simulink model "Torque_Mode_OpenLoop"  (R2014a)
settings: Solver=ode5  StartTime=0.0  StopTime=T_f+0.1  FixedStep=0.001  RelTol=1e-3
InitFcn:
  | load('New_Demo')
  | T_f=37;
undefined symbols (not defined in the file or in its folder): Standard_Devices, UDP_Protocol
libraries: simulink x4, rtwinlib x3, slrtlib x1
(part 1 of 2)
settings Model: SimulationMode=external  ExtModeTrigDuration=70000  ExtModeTrigDurationFloating=70000  Creator=user  LastModifiedBy=user
settings HardwareCC: ProdIntDivRoundTo=Zero  ProdEndianess=LittleEndian  ProdHWDeviceType=Generic->32-bit x86 compatible
settings RTWCC: SystemTargetFile=rtwin.tlc  TemplateMakefile=rtwin.tmf  Description=Real-Time Windows Target  ProcessScript=rtwin_make_rtw_hook  RTWCompilerOptimization=On
settings CodeAppCC: MaxIdLength=95
settings RTWinTargetCC: TargetLibSuffix=_rtwin.lib  TargetPreCompLibLocation=C:\Program Files\MATLAB\R2014a\toolbox\rtw\targets\rtwin\lib\win64

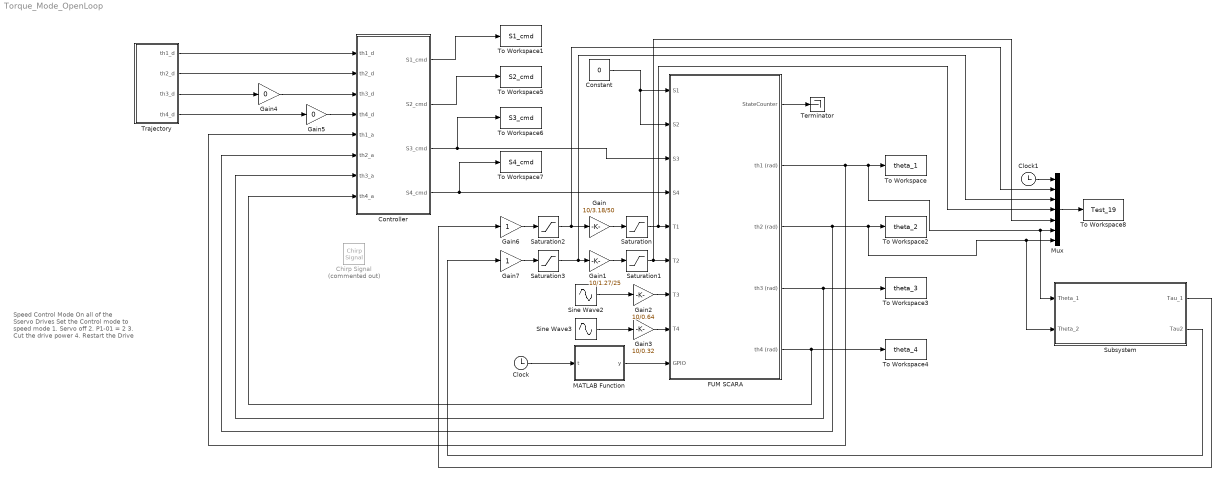
== system Torque_Mode_OpenLoop ==
  note: Speed Control Mode
      | On all of the Sservo Drives Set the
      | Control mode to speed mode
      | 1. Servo off
      | 2. P1-01 = 2
      | 3. Cut the drive power
      | 4. Restart the Drive
  Chirp Signal : simulink/Sources/Chirp Signal  Commented=on  f1=1/2/pi  T=T_f  f2=5/2/pi
  Clock : Clock
      settings: Decimation=20
  Clock1 : Clock
  Constant : Constant  Value=0
  Controller : Subsystem
  FUM SCARA : Subsystem
  Gain : Gain  Gain=10/3.18/50
  Gain1 : Gain  Gain=10/1.27/25
  Gain2 : Gain  Gain=10/0.64
  Gain3 : Gain  Gain=10/0.32
  Gain4 : Gain  Gain=0
  Gain5 : Gain  Gain=0
  Gain6 : Gain
  Gain7 : Gain
  MATLAB Function : MATLAB Function  TreatAsAtomicUnit=on
  Mux : Mux  Inputs=7
  Saturation : Saturate  UpperLimit=5  LowerLimit=-5
  Saturation1 : Saturate  UpperLimit=5  LowerLimit=-5
  Saturation2 : Saturate  UpperLimit=30  LowerLimit=-30
  Saturation3 : Saturate  UpperLimit=10  LowerLimit=-10
  Sine Wave2 : Sin  Amplitude=0  SampleTime=0
  Sine Wave3 : Sin  Amplitude=0  SampleTime=0
  Subsystem : Subsystem
  Terminator : Terminator
  To Workspace : ToWorkspace  VariableName=theta_1  SampleTime=-1
  To Workspace1 : ToWorkspace  VariableName=S1_cmd  SampleTime=-1
  To Workspace2 : ToWorkspace  VariableName=theta_2  SampleTime=-1
  To Workspace3 : ToWorkspace  VariableName=theta_3  SampleTime=-1
  To Workspace4 : ToWorkspace  VariableName=theta_4  SampleTime=-1
  To Workspace5 : ToWorkspace  VariableName=S2_cmd  SampleTime=-1
  To Workspace6 : ToWorkspace  VariableName=S3_cmd  SampleTime=-1
  To Workspace7 : ToWorkspace  VariableName=S4_cmd  SampleTime=-1
  To Workspace8 : ToWorkspace  VariableName=Test_19  SampleTime=-1
  Trajectory : Subsystem
  wires:
  FUM SCARA/1(StateCounter) -> Terminator/1
  Trajectory/1(th1_d) -> Controller/1(th1_d)
  Trajectory/2(th2_d) -> Controller/2(th2_d)
  Trajectory/3(th3_d) -> Gain4/1
  Trajectory/4(th4_d) -> Gain5/1
  FUM SCARA/5(th4 (rad)) -> Controller/8(th4_a), To Workspace4/1
  FUM SCARA/4(th3 (rad)) -> Controller/7(th3_a), To Workspace3/1
  FUM SCARA/3(th2 (rad)) -> Controller/6(th2_a), Subsystem/2(Theta_2), Mux/7, To Workspace2/1
  FUM SCARA/2(th1 (rad)) -> Controller/5(th1_a), Subsystem/1(Theta_1), Mux/6, To Workspace/1
  Clock/1 -> MATLAB Function/1(t)
  MATLAB Function/1(y) -> FUM SCARA/9(GPIO)
  Controller/1(S1_cmd) -> To Workspace1/1
  Controller/2(S2_cmd) -> To Workspace5/1
  Controller/3(S3_cmd) -> To Workspace6/1, FUM SCARA/3(S3)
  Controller/4(S4_cmd) -> FUM SCARA/4(S4), To Workspace7/1
  Constant/1 -> FUM SCARA/2(S2), FUM SCARA/1(S1)
  Sine Wave2/1 -> Gain2/1
  Sine Wave3/1 -> Gain3/1
  Gain/1 -> Saturation/1
  Gain1/1 -> Saturation1/1
  Gain2/1 -> FUM SCARA/7(T3)
  Gain3/1 -> FUM SCARA/8(T4)
  Gain4/1 -> Controller/3(th3_d)
  Gain5/1 -> Controller/4(th4_d)
  Gain6/1 -> Saturation2/1
  Gain7/1 -> Saturation3/1
  Saturation/1 -> Mux/4, FUM SCARA/5(T1)
  Saturation1/1 -> FUM SCARA/6(T2), Mux/5
  Clock1/1 -> Mux/1
  Mux/1 -> To Workspace8/1
  Subsystem/2(Tau2) -> Gain7/1
  Subsystem/1(Tau_1) -> Gain6/1
  Saturation2/1 -> Gain/1, Mux/2
  Saturation3/1 -> Mux/3, Gain1/1

== system Torque_Mode_OpenLoop/Controller ==
  th1_d : Inport
  th2_d : Inport  Port=2
  th3_d : Inport  Port=3
  th4_d : Inport  Port=4
  th1_a : Inport  Port=5
  th2_a : Inport  Port=6
  th3_a : Inport  Port=7
  th4_a : Inport  Port=8
  Gain10 : Gain  Gain=0.25  SampleTime=0.001
  Gain16 : Gain  Gain=0.5  SampleTime=0.001
  Gain5 : Gain  Gain=0.5  SampleTime=0.001
  Gain9 : Gain  Gain=0.4  SampleTime=0.001
  Sum{2,5..6,8} (4 alike) : Sum  Inputs=|+-
  S1_cmd : Outport
  S2_cmd : Outport  Port=2
  S3_cmd : Outport  Port=3
  S4_cmd : Outport  Port=4
  wires:
  th2_a/1 -> Sum2/2
  Sum2/1 -> Gain5/1
  th3_a/1 -> Sum5/2
  Sum5/1 -> Gain10/1
  Sum8/1 -> Gain16/1
  th1_a/1 -> Sum6/2
  th4_a/1 -> Sum8/2
  Sum6/1 -> Gain9/1
  Gain16/1 -> S4_cmd/1
  Gain9/1 -> S1_cmd/1
  Gain5/1 -> S2_cmd/1
  Gain10/1 -> S3_cmd/1
  th2_d/1 -> Sum2/1
  th3_d/1 -> Sum5/1
  th1_d/1 -> Sum6/1
  th4_d/1 -> Sum8/1

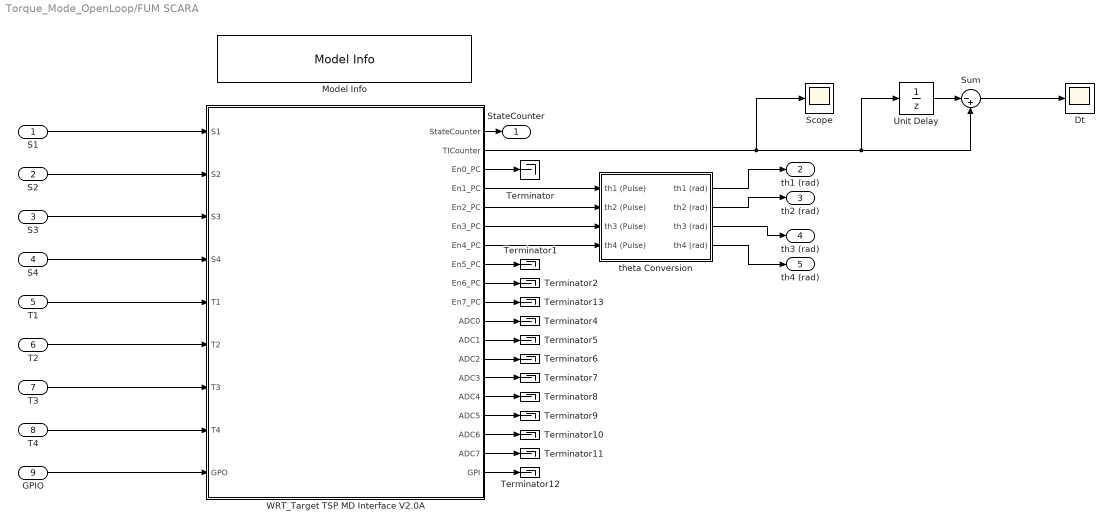
== system Torque_Mode_OpenLoop/FUM SCARA ==
  S1 : Inport
  S2 : Inport  Port=2
  S3 : Inport  Port=3
  S4 : Inport  Port=4
  T1 : Inport  Port=5
  T2 : Inport  Port=6
  T3 : Inport  Port=7
  T4 : Inport  Port=8
  GPIO : Inport  Port=9
  Dt : Scope
      settings: TimeRange=7  YMin=0  YMax=2  SaveName=Dt
  Model Info : simulink/Model-Wide Utilities/Model Info  InitialBlockCM=None  BlockCM=None  Frame=on  DisplayStringWithTags="TSP MD Interface With Windows  Real Time Target"  HorizontalTextAlignment=Center  LeftAlignmentValue=0.5  SourceBlockDiagram=Torque_Mode_OpenLoop  TagMaxNumber=20
  Scope : Scope
      settings: TimeRange=60  YMin=0  YMax=275
  Sum : Sum  Inputs=|-+
  Terminator{,1..2,4..13} (13 alike) : Terminator
  Unit Delay : UnitDelay  SampleTime=-1
  WRT_Target TSP MD Interface V2.0A : Subsystem  mask(TSP MDI Send UDP Packet){SampleTime=0.001, MaxProcTime=T_f*1000, ADC_Mode=8 Single-Ended Inputs, ADC_Range=± 10 V}
      mask prompts: SampleTime "Sample Time"; MaxProcTime "Total Processing Counter"; ADC_Mode "ADC Mode"; ADC_Range "ADC Range"
      mask help: This Block Manage Sending UDP Packet To TSP MDI Board
      mask TypeOptions ADC_Mode: 8 Single-Ended Inputs | 4 Pseudo Differential Inputs | 4 Fully Differential Inputs | Pseudo Differential Inputs
      mask TypeOptions ADC_Range: ± 10 V | ± 5 V | ± 2.5 V | 0-10 V
  theta Conversion : Subsystem
  StateCounter : Outport
  th1 (rad) : Outport  Port=2
  th2 (rad) : Outport  Port=3
  th3 (rad) : Outport  Port=4
  th4 (rad) : Outport  Port=5
  wires:
  WRT_Target TSP MD Interface V2.0A/1(StateCounter) -> StateCounter/1
  WRT_Target TSP MD Interface V2.0A/2(TICounter) -> Scope/1, Unit Delay/1, Sum/2
  theta Conversion/1(th1 (rad)) -> th1 (rad)/1
  theta Conversion/3(th3 (rad)) -> th3 (rad)/1
  theta Conversion/4(th4 (rad)) -> th4 (rad)/1
  Unit Delay/1 -> Sum/1
  WRT_Target TSP MD Interface V2.0A/4(En1_PC) -> theta Conversion/1(th1 (Pulse))
  WRT_Target TSP MD Interface V2.0A/5(En2_PC) -> theta Conversion/2(th2 (Pulse))
  WRT_Target TSP MD Interface V2.0A/6(En3_PC) -> theta Conversion/3(th3 (Pulse))
  WRT_Target TSP MD Interface V2.0A/3(En0_PC) -> Terminator/1
  WRT_Target TSP MD Interface V2.0A/8(En5_PC) -> Terminator1/1
  WRT_Target TSP MD Interface V2.0A/9(En6_PC) -> Terminator2/1
  WRT_Target TSP MD Interface V2.0A/11(ADC0) -> Terminator4/1
  WRT_Target TSP MD Interface V2.0A/12(ADC1) -> Terminator5/1
  WRT_Target TSP MD Interface V2.0A/13(ADC2) -> Terminator6/1
  WRT_Target TSP MD Interface V2.0A/14(ADC3) -> Terminator7/1
  WRT_Target TSP MD Interface V2.0A/15(ADC4) -> Terminator8/1
  WRT_Target TSP MD Interface V2.0A/16(ADC5) -> Terminator9/1
  WRT_Target TSP MD Interface V2.0A/17(ADC6) -> Terminator10/1
  WRT_Target TSP MD Interface V2.0A/18(ADC7) -> Terminator11/1
  WRT_Target TSP MD Interface V2.0A/19(GPI) -> Terminator12/1
  Sum/1 -> Dt/1
  WRT_Target TSP MD Interface V2.0A/7(En4_PC) -> theta Conversion/4(th4 (Pulse))
  WRT_Target TSP MD Interface V2.0A/10("En7_PC ") -> Terminator13/1
  theta Conversion/2(th2 (rad)) -> th2 (rad)/1
  S1/1 -> WRT_Target TSP MD Interface V2.0A/1(S1)
  S2/1 -> WRT_Target TSP MD Interface V2.0A/2(S2)
  S3/1 -> WRT_Target TSP MD Interface V2.0A/3(S3)
  S4/1 -> WRT_Target TSP MD Interface V2.0A/4(S4)
  GPIO/1 -> WRT_Target TSP MD Interface V2.0A/9(GPO)
  T1/1 -> WRT_Target TSP MD Interface V2.0A/5(T1)
  T2/1 -> WRT_Target TSP MD Interface V2.0A/6(T2)
  T3/1 -> WRT_Target TSP MD Interface V2.0A/7(T3)
  T4/1 -> WRT_Target TSP MD Interface V2.0A/8(T4)

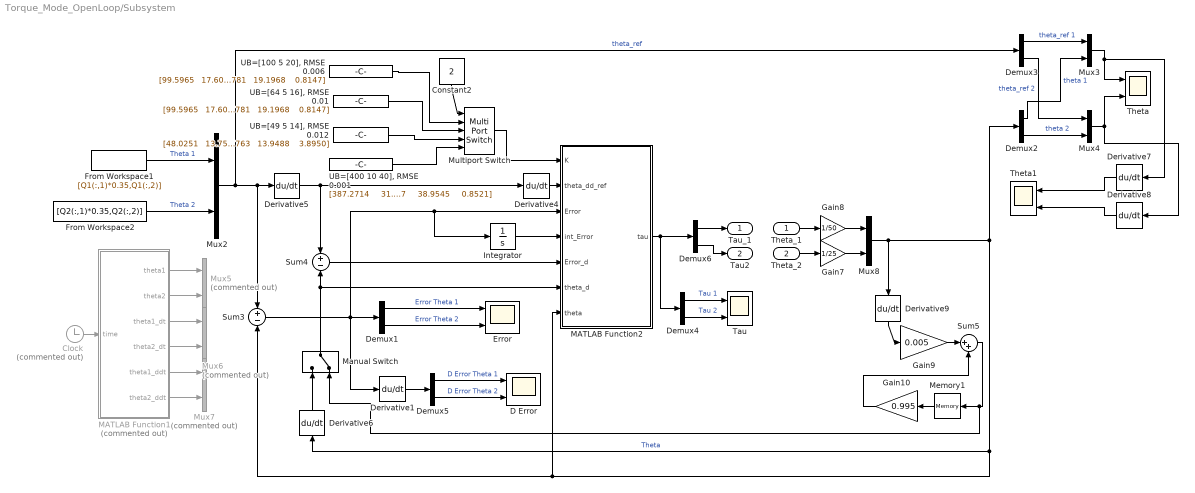
== system Torque_Mode_OpenLoop/Subsystem ==
  Theta_1 : Inport
  Theta_2 : Inport  Port=2
  Clock : Clock  Commented=on
  Constant2 : Constant  Value=2
  D Error : Scope  NumInputPorts=2
      settings: ShowLegends=on  YMin=-0.13078~-0.07305  YMax=0.12037~0.07273  SaveName=ScopeData3
  Demux{1..6} (6 alike) : Demux  Outputs=2
  Derivative{1,4..9} (7 alike) : Derivative
  Error : Scope  NumInputPorts=2
      settings: ShowLegends=on  YMin=-0.00785~-0.01145  YMax=-0.00764~-0.011175  SaveName=ScopeData4
  From Workspace1 : FromWorkspace  VariableName=[Q1(:,1)*0.35,Q1(:,2)]  SampleTime=0
  From Workspace2 : FromWorkspace  VariableName=[Q2(:,1)*0.35,Q2(:,2)]  SampleTime=0
  Gain10 : Gain  Gain=0.995
  Gain7 : Gain  Gain=1/25
  Gain8 : Gain  Gain=1/50
  Gain9 : Gain  Gain=0.005
  Integrator : Integrator
  MATLAB Function1 : MATLAB Function  Commented=on  TreatAsAtomicUnit=on
  MATLAB Function2 : MATLAB Function  TreatAsAtomicUnit=on
  Manual Switch : ManualSwitch  CurrentSetting=0
  Memory1 : Memory
  Multiport Switch : MultiPortSwitch  Inputs=4
  Mux{2..4,8} (4 alike) : Mux  Inputs=2
  Mux5 : Mux  Commented=on  Inputs=2
  Mux6 : Mux  Commented=on  Inputs=2
  Mux7 : Mux  Commented=on  Inputs=2
  Sum3 : Sum  Inputs=+|-
  Sum4 : Sum  Inputs=+|-
  Sum5 : Sum  Inputs=|++
  Tau : Scope  NumInputPorts=2
      settings: ShowLegends=on  YMin=50~0  YMax=550~105  SaveName=ScopeData5
  Theta : Scope  NumInputPorts=2
      settings: ShowLegends=on  YMin=-0.0025~-0.0025  YMax=0.035~0.025  SaveName=ScopeData6
  Theta1 : Scope  NumInputPorts=2
      settings: ShowLegends=on  YMin=-0.49087~-0.49093  YMax=0.49087~0.49136  SaveName=ScopeData7
  "UB=[100 5 20], RMSE 0.006" : Constant  Value="[99.5965   17.6001    3.0916   96.6781   19.1968    0.8147]"
  "UB=[400 10 40], RMSE 0.001" : Constant  Value="[387.2714     31.6242     8.5375     369.6227     38.9545     0.8521]"
  "UB=[49 5 14], RMSE 0.012" : Constant  Value="[48.0251   13.7536    2.4862   48.4763   13.9488    3.8950]"
  "UB=[64 5 16], RMSE 0.01" : Constant  Value="[99.5965   17.6001    3.0916   96.6781   19.1968    0.8147]"
  Tau_1 : Outport
  Tau2 : Outport  Port=2
  wires:
  Sum3/1 -> Demux1/1, Derivative1/1, Integrator/1, MATLAB Function2/3(Error)
  MATLAB Function2/1(tau) -> Demux6/1, Demux4/1
  Mux8/1 -> Derivative9/1, Demux2/1, Derivative6/1, MATLAB Function2/7(theta), Sum3/2  "Theta"
  Sum5/1 -> Manual Switch/2, Memory1/1
  Demux1/2 -> Error/2  "Error Theta 2"
  Demux1/1 -> Error/1  "Error Theta 1"
  Mux3/1 -> Theta/1, Derivative7/1
  Mux4/1 -> Theta/2, Derivative8/1
  Demux2/1 -> Mux3/2  "theta 1"
  Demux3/1 -> Mux3/1  "theta_ref 1"
  Demux2/2 -> Mux4/2  "theta 2"
  Demux3/2 -> Mux4/1  "theta_ref 2"
  Integrator/1 -> MATLAB Function2/4(int_Error)
  Sum4/1 -> MATLAB Function2/5(Error_d)
  From Workspace2/1 -> Mux2/2  "Theta 2"
  From Workspace1/1 -> Mux2/1  "Theta 1"
  Demux4/1 -> Tau/1  "Tau 1"
  Demux4/2 -> Tau/2  "Tau 2"
  Demux5/1 -> D Error/1  "D Error Theta 1"
  Demux5/2 -> D Error/2  "D Error Theta 2"
  Derivative1/1 -> Demux5/1
  "UB=[100 5 20], RMSE 0.006"/1 -> Multiport Switch/2
  Constant2/1 -> Multiport Switch/1
  "UB=[64 5 16], RMSE 0.01"/1 -> Multiport Switch/3
  Clock/1 -> MATLAB Function1/1(time)
  MATLAB Function1/1(theta1) -> Mux5/1
  MATLAB Function1/2(theta2) -> Mux5/2
  MATLAB Function1/5(theta1_ddt) -> Mux7/1
  MATLAB Function1/6(theta2_ddt) -> Mux7/2
  MATLAB Function1/4(theta2_dt) -> Mux6/2
  MATLAB Function1/3(theta1_dt) -> Mux6/1
  "UB=[49 5 14], RMSE 0.012"/1 -> Multiport Switch/4
  Derivative4/1 -> MATLAB Function2/2(theta_dd_ref)
  Mux2/1 -> Derivative5/1, Sum3/1, Demux3/1  "theta_ref"
  Derivative5/1 -> Sum4/1, Derivative4/1
  Derivative7/1 -> Theta1/1
  Derivative8/1 -> Theta1/2
  Demux6/2 -> Tau2/1
  Theta_1/1 -> Gain8/1
  Demux6/1 -> Tau_1/1
  Gain8/1 -> Mux8/1
  Gain7/1 -> Mux8/2
  Theta_2/1 -> Gain7/1
  Memory1/1 -> Gain10/1
  Gain10/1 -> Sum5/2
  Gain9/1 -> Sum5/1
  Manual Switch/1 -> MATLAB Function2/6(theta_d), Sum4/2
  Derivative6/1 -> Manual Switch/1
  Derivative9/1 -> Gain9/1
  Multiport Switch/1 -> MATLAB Function2/1(K)
  "UB=[400 10 40], RMSE 0.001"/1 -> Multiport Switch/5

== system Torque_Mode_OpenLoop/Trajectory ==
  Demux1 : Demux  Outputs=12
  From Workspace : FromWorkspace  VariableName=trajectory  SampleTime=0  OutputAfterFinalValue=Holding final value
  Gain{4,8,15,19} (4 alike) : Gain
  Terminator{1..8} (8 alike) : Terminator
  To Workspace : ToWorkspace  VariableName=th1_d  SampleTime=-1
  To Workspace1 : ToWorkspace  VariableName=th2_d  SampleTime=-1
  To Workspace2 : ToWorkspace  VariableName=th3_d  SampleTime=-1
  To Workspace3 : ToWorkspace  VariableName=th4_d  SampleTime=-1
  th1_d : Outport
  th2_d : Outport  Port=2
  th3_d : Outport  Port=3
  th4_d : Outport  Port=4
  wires:
  Demux1/7 -> Gain15/1
  Demux1/10 -> Gain19/1
  Demux1/4 -> Gain8/1
  Gain15/1 -> To Workspace2/1, th3_d/1
  Gain19/1 -> To Workspace3/1, th4_d/1
  Gain8/1 -> To Workspace1/1, th2_d/1
  Gain4/1 -> To Workspace/1, th1_d/1
  From Workspace/1 -> Demux1/1
  Demux1/1 -> Gain4/1
  Demux1/5 -> Terminator3/1
  Demux1/8 -> Terminator5/1
  Demux1/12 -> Terminator8/1
  Demux1/6 -> Terminator4/1
  Demux1/3 -> Terminator2/1
  Demux1/2 -> Terminator1/1
  Demux1/11 -> Terminator7/1
  Demux1/9 -> Terminator6/1

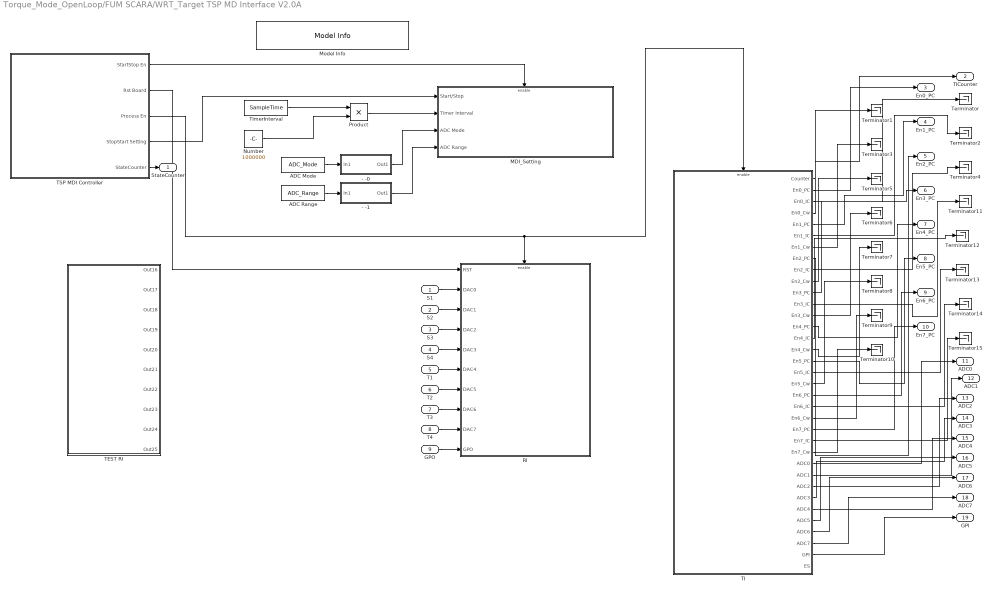
== system Torque_Mode_OpenLoop/FUM SCARA/WRT_Target TSP MD Interface V2.0A ==
  S1 : Inport
  S2 : Inport  Port=2
  S3 : Inport  Port=3
  S4 : Inport  Port=4
  T1 : Inport  Port=5
  T2 : Inport  Port=6
  T3 : Inport  Port=7
  T4 : Inport  Port=8
  GPO : Inport  Port=9
  - -0 : Subsystem
  - -1 : Subsystem
  ADC Mode : Constant  Value=ADC_Mode  SampleTime=-1
  ADC Range : Constant  Value=ADC_Range  SampleTime=-1
  MDI_Setting : Subsystem  TreatAsAtomicUnit=on  mask(Setting UDP Packet Sender){HostMAC=[255 255 255 255 255 255], DeviceMAC=[11 12 13 14 15 16], HostIP1=192, HostIP2=168, HostIP3=1, HostIP4=100, DeviceIP1=192, DeviceIP2=168, DeviceIP3=1, DeviceIP4=22, HostPort=[23000], DevicePort=[23001], SampleTime=SampleTime}
      mask prompts: HostMAC "Host Mac"; DeviceMAC "Device Mac"; HostPort "Host Port"; DevicePort "Device Port"; SampleTime "Sample Time"
      mask help: This Block Genetate And Send UDP Packet To MDI TSP Board For Setting Board
      settings: PropExecContextOutsideSubsystem=on
      mask DialogControl Container10 Prompt: HOST IP
      mask DialogControl Container11 Prompt: DEVICE IP
  Model Info : simulink/Model-Wide Utilities/Model Info  InitialBlockCM=None  BlockCM=None  Frame=on  DisplayStringWithTags=TSP MDI Board With Windows Real Time Target  HorizontalTextAlignment=Center  LeftAlignmentValue=0.5  SourceBlockDiagram=Torque_Mode_OpenLoop  TagMaxNumber=20
  Number : Constant  Value=1000000  SampleTime=-1
  Product : Product
  RI : Subsystem  mask(Receive Informations Packet Generator){En0_e=on, En1_e=on, En2_e=on, En4_e=on, En3_e=on, En5_e=on, En6_e=on, En7_e=on, SampleTime=SampleTime}
      mask prompts: En0_e "Encoder 0 Enable"; En1_e "Encoder 1 Enable"; En2_e "Encoder 2 Enable"; En4_e "Encoder 4 Enable"; En3_e "Encoder 3 Enable"; En5_e "Encoder 5 Enable"; En6_e "Encoder 6 Enable"; En7_e "Encoder 7 Enable"; SampleTime "Sample Time"
      mask DialogControl Control2 Prompt: This Block Generate And Send Receive Informations UDP Packet To MDI TSP Board
  TEST RI : Subsystem
  TI : Subsystem  mask(Receive Information UDP Packet Receiver){SampleTime=SampleTime}
      mask prompts: SampleTime "Sample Time"
      mask help: This Block Receive And Extract Transmit Information UDP Packet From MDI TSP Board
  TSP MDI Controller : Subsystem  mask(TSP MDI Controller){}
      mask help: This Block Controll TSP MDI Board
      mask Help: Set Maximum Count For Time Processing
  Terminator{,1..15} (16 alike) : Terminator
  TimerInterval : Constant  Value=SampleTime  SampleTime=-1
  StateCounter : Outport
  TICounter : Outport  Port=2
  En0_PC : Outport  Port=3
  En1_PC : Outport  Port=4
  En2_PC : Outport  Port=5
  En3_PC : Outport  Port=6
  En4_PC : Outport  Port=7
  En5_PC : Outport  Port=8
  En6_PC : Outport  Port=9
  "En7_PC " : Outport  Port=10
  ADC0 : Outport  Port=11
  ADC1 : Outport  Port=12
  ADC2 : Outport  Port=13
  ADC3 : Outport  Port=14
  ADC4 : Outport  Port=15
  ADC5 : Outport  Port=16
  ADC6 : Outport  Port=17
  ADC7 : Outport  Port=18
  GPI : Outport  Port=19
  wires:
  TI/1(Counter) -> TICounter/1
  TSP MDI Controller/1(StartStop En) -> MDI_Setting/Enable
  TimerInterval/1 -> Product/1
  Number/1 -> Product/2
  Product/1 -> MDI_Setting/2(Timer Interval)
  TI/2(En0_PC) -> En0_PC/1
  TI/5(En1_PC) -> En1_PC/1
  TI/8(En2_PC) -> En2_PC/1
  TI/11(En3_PC) -> En3_PC/1
  TSP MDI Controller/4(StopStart Setting) -> MDI_Setting/1(Start/Stop)
  TSP MDI Controller/3(Process En) -> TI/Enable, RI/Enable
  TSP MDI Controller/5(StateCounter) -> StateCounter/1
  ADC Mode/1 -> - -0/1(In1)
  ADC Range/1 -> - -1/1(In1)
  - -0/1(Out1) -> MDI_Setting/3(ADC Mode)
  - -1/1(Out1) -> MDI_Setting/4(ADC Range)
  TI/26(ADC0) -> ADC0/1
  TI/28(ADC2) -> ADC2/1
  TI/29(ADC3) -> ADC3/1
  TI/30(ADC4) -> ADC4/1
  TI/31(ADC5) -> ADC5/1
  TI/32(ADC6) -> ADC6/1
  TI/33(ADC7) -> ADC7/1
  TI/34(GPI) -> GPI/1
  TI/3(En0_IC) -> Terminator/1
  TI/6(En1_IC) -> Terminator2/1
  TI/9(En2_IC) -> Terminator4/1
  TI/12(En3_IC) -> Terminator11/1
  TI/14(En4_PC) -> En4_PC/1
  TI/15(En4_IC) -> Terminator12/1
  TI/17(En5_PC) -> En5_PC/1
  TI/18(En5_IC) -> Terminator13/1
  TI/20(En6_PC) -> En6_PC/1
  TI/21(En6_IC) -> Terminator14/1
  TI/23(En7_PC) -> "En7_PC "/1
  TI/24(En7_IC) -> Terminator15/1
  TI/4(En0_Cw) -> Terminator1/1
  TI/7(En1_Cw) -> Terminator3/1
  TI/10(En2_Cw) -> Terminator5/1
  TI/13(En3_Cw) -> Terminator6/1
  TI/16(En4_Cw) -> Terminator7/1
  TI/19(En5_Cw) -> Terminator8/1
  TI/22(En6_Cw) -> Terminator9/1
  TI/25(En7_Cw) -> Terminator10/1
  TI/27(ADC1) -> ADC1/1
  GPO/1 -> RI/10(GPO)
  TSP MDI Controller/2(Rst Board) -> RI/1(RST)
  T4/1 -> RI/9(DAC7)
  T3/1 -> RI/8(DAC6)
  T2/1 -> RI/7(DAC5)
  T1/1 -> RI/6(DAC4)
  S1/1 -> RI/2(DAC0)
  S2/1 -> RI/3(DAC1)
  S3/1 -> RI/4(DAC2)
  S4/1 -> RI/5(DAC3)

== system Torque_Mode_OpenLoop/FUM SCARA/theta Conversion ==
  th1 (Pulse) : Inport
  th2 (Pulse) : Inport  Port=2
  th3 (Pulse) : Inport  Port=3
  th4 (Pulse) : Inport  Port=4
  Data Type Conversion{,1..3} (4 alike) : DataTypeConversion  SampleTime=0.001
  Gain{1..2,6,9} (4 alike) : Gain  Gain=1/160000
  Gain{3,7,10,12} (4 alike) : Gain  Gain=2*pi
  Gain{4..5,8,11} (4 alike) : Gain  Gain=-1
  th1 (rad) : Outport
  th2 (rad) : Outport  Port=2
  th3 (rad) : Outport  Port=3
  th4 (rad) : Outport  Port=4
  wires:
  th2 (Pulse)/1 -> Gain2/1
  Gain10/1 -> th4 (rad)/1
  Data Type Conversion3/1 -> Gain11/1
  Gain12/1 -> th1 (rad)/1
  th3 (Pulse)/1 -> Gain6/1
  Data Type Conversion1/1 -> Gain5/1
  th4 (Pulse)/1 -> Gain9/1
  Data Type Conversion2/1 -> Gain8/1
  Gain7/1 -> th3 (rad)/1
  Gain9/1 -> Data Type Conversion3/1
  Gain3/1 -> th2 (rad)/1
  Gain2/1 -> Data Type Conversion1/1
  Gain6/1 -> Data Type Conversion2/1
  Data Type Conversion/1 -> Gain4/1
  Gain1/1 -> Data Type Conversion/1
  th1 (Pulse)/1 -> Gain1/1
  Gain4/1 -> Gain12/1
  Gain5/1 -> Gain3/1
  Gain8/1 -> Gain7/1
  Gain11/1 -> Gain10/1

== system Torque_Mode_OpenLoop/FUM SCARA/WRT_Target TSP MD Interface V2.0A/- -0 ==
  In1 : Inport
  Constant2 : Constant
  Sum : Sum  Inputs=|+-
  Out1 : Outport
  wires:
  In1/1 -> Sum/1
  Sum/1 -> Out1/1
  Constant2/1 -> Sum/2

== system Torque_Mode_OpenLoop/FUM SCARA/WRT_Target TSP MD Interface V2.0A/- -1 ==
  In1 : Inport
  Constant2 : Constant
  Sum : Sum  Inputs=|+-
  Out1 : Outport
  wires:
  In1/1 -> Sum/1
  Sum/1 -> Out1/1
  Constant2/1 -> Sum/2

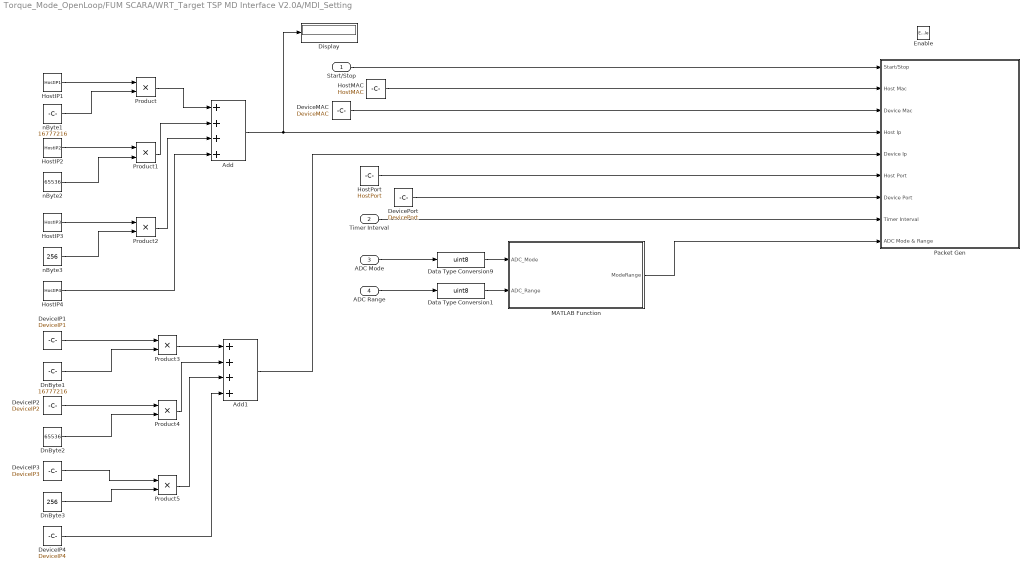
== system Torque_Mode_OpenLoop/FUM SCARA/WRT_Target TSP MD Interface V2.0A/MDI_Setting ==
  Start/Stop : Inport
  Timer Interval : Inport  Port=2
  ADC Mode : Inport  Port=3
  ADC Range : Inport  Port=4
  Enable : EnablePort
  Add : Sum  Inputs=++++
  Add1 : Sum  Inputs=++++
  Data Type Conversion1 : DataTypeConversion  OutDataTypeStr=uint8
  Data Type Conversion9 : DataTypeConversion  OutDataTypeStr=uint8
  DeviceIP1 : Constant  Value=DeviceIP1  SampleTime=-1
  DeviceIP2 : Constant  Value=DeviceIP2  SampleTime=-1
  DeviceIP3 : Constant  Value=DeviceIP3  SampleTime=-1
  DeviceIP4 : Constant  Value=DeviceIP4  SampleTime=-1
  DeviceMAC : Constant  Value=DeviceMAC  SampleTime=-1
  DevicePort : Constant  Value=DevicePort  SampleTime=-1
  Display : Display
  DnByte1 : Constant  Value=16777216
  DnByte2 : Constant  Value=65536  SampleTime=-1
  DnByte3 : Constant  Value=256  SampleTime=-1
  HostIP1 : Constant  Value=HostIP1  SampleTime=-1
  HostIP2 : Constant  Value=HostIP2  SampleTime=-1
  HostIP3 : Constant  Value=HostIP3  SampleTime=-1
  HostIP4 : Constant  Value=HostIP4  SampleTime=-1
  HostMAC : Constant  Value=HostMAC  SampleTime=-1
  HostPort : Constant  Value=HostPort  SampleTime=-1
  MATLAB Function : MATLAB Function  TreatAsAtomicUnit=on
  Packet Gen : Subsystem
  Product{,1..5} (6 alike) : Product
  nByte1 : Constant  Value=16777216
  nByte2 : Constant  Value=65536  SampleTime=-1
  nByte3 : Constant  Value=256  SampleTime=-1
  wires:
  Start/Stop/1 -> Packet Gen/1(Start/Stop)
  HostMAC/1 -> Packet Gen/2(Host Mac)
  DeviceMAC/1 -> Packet Gen/3(Device Mac)
  HostPort/1 -> Packet Gen/6(Host Port)
  DevicePort/1 -> Packet Gen/7(Device Port)
  Timer Interval/1 -> Packet Gen/8(Timer Interval)
  HostIP1/1 -> Product/1
  nByte1/1 -> Product/2
  HostIP2/1 -> Product1/1
  nByte2/1 -> Product1/2
  HostIP3/1 -> Product2/1
  nByte3/1 -> Product2/2
  Product/1 -> Add/1
  Product1/1 -> Add/2
  Product2/1 -> Add/3
  HostIP4/1 -> Add/4
  DeviceIP1/1 -> Product3/1
  DnByte1/1 -> Product3/2
  DeviceIP2/1 -> Product4/1
  DnByte2/1 -> Product4/2
  DeviceIP3/1 -> Product5/1
  DnByte3/1 -> Product5/2
  Product3/1 -> Add1/1
  Product4/1 -> Add1/2
  Product5/1 -> Add1/3
  DeviceIP4/1 -> Add1/4
  Add1/1 -> Packet Gen/5(Device Ip)
  Data Type Conversion9/1 -> MATLAB Function/1(ADC_Mode)
  Data Type Conversion1/1 -> MATLAB Function/2(ADC_Range)
  ADC Mode/1 -> Data Type Conversion9/1
  ADC Range/1 -> Data Type Conversion1/1
  MATLAB Function/1(ModeRange) -> Packet Gen/9(ADC Mode & Range)
  Add/1 -> Display/1, Packet Gen/4(Host Ip)

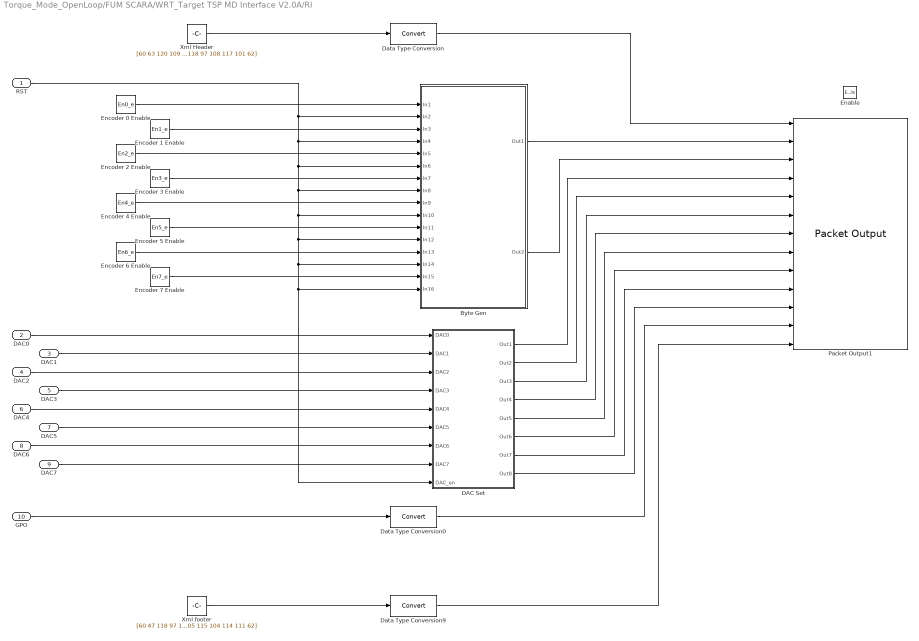
== system Torque_Mode_OpenLoop/FUM SCARA/WRT_Target TSP MD Interface V2.0A/RI ==
  RST : Inport
  DAC0 : Inport  Port=2
  DAC1 : Inport  Port=3
  DAC2 : Inport  Port=4
  DAC3 : Inport  Port=5
  DAC4 : Inport  Port=6
  DAC5 : Inport  Port=7
  DAC6 : Inport  Port=8
  DAC7 : Inport  Port=9
  GPO : Inport  Port=10
  Enable : EnablePort
  Byte Gen : Subsystem
  DAC Set : Subsystem
  Data Type Conversion : DataTypeConversion
  Data Type Conversion0 : DataTypeConversion
  Data Type Conversion9 : DataTypeConversion
  Encoder 0 Enable : Constant  Value=En0_e
  Encoder 1 Enable : Constant  Value=En1_e
  Encoder 2 Enable : Constant  Value=En2_e
  Encoder 3 Enable : Constant  Value=En3_e
  Encoder 4 Enable : Constant  Value=En4_e
  Encoder 5 Enable : Constant  Value=En5_e
  Encoder 6 Enable : Constant  Value=En6_e
  Encoder 7 Enable : Constant  Value=En7_e
  Packet Output1 : rtwinlib/Packet Output  SampleTime=SampleTime  MaxMissedTicks=1000  ShowMissedTicks=off  YieldWhenWaiting=on  DrvName=Standard_Devices/UDP_Protocol  DrvAddress=100  DrvOptions=[3232236031 101]  PacketSize=117  DataTypes={'78*uint8','uint8','uint8','uint16','uint16','uint16','uint16','uint16','uint16','uint16','uint16','uint16','19*uint8'}  ShowReady=off  ShowError=off  PacketID=1  ByteOrder=1  InitialValue=[]  FinalValue=[]
      settings: AttributesFormatString=Standard Devices\nUDP Protocol [64h]
  Xml Header : Constant  Value="[60 63 120 109 108 32 118 101 114 115 105 111 110 61 34  49 46 48 34 63 62 60 116 115 112 105 115 104 114 111 62 60 116 121 112 101 62 114 101 99 101 105 118 101 95 105 110 102 111 60 47 116 121 112 101 62 60 115 105 122 101 62 50 48 60 47 115 105 122 101 62 60 118 97 108 117 101 62]"  LockScale=on
  Xml footer : Constant  Value=[60 47 118 97 108 117 101 62 60 47 116 115 112 105 115 104 114 111 62]
  wires:
  Xml Header/1 -> Data Type Conversion/1
  Xml footer/1 -> Data Type Conversion9/1
  Data Type Conversion/1 -> Packet Output1/1
  Data Type Conversion9/1 -> Packet Output1/13
  Encoder 0 Enable/1 -> Byte Gen/1(In1)
  Encoder 1 Enable/1 -> Byte Gen/3(In3)
  Encoder 2 Enable/1 -> Byte Gen/5(In5)
  Encoder 3 Enable/1 -> Byte Gen/7(In7)
  Encoder 4 Enable/1 -> Byte Gen/9(In9)
  Encoder 6 Enable/1 -> Byte Gen/13(In13)
  Encoder 7 Enable/1 -> Byte Gen/15(In15)
  GPO/1 -> Data Type Conversion0/1
  Data Type Conversion0/1 -> Packet Output1/12
  Byte Gen/1(Out1) -> Packet Output1/2
  Byte Gen/2(Out2) -> Packet Output1/3
  Encoder 5 Enable/1 -> Byte Gen/11(In11)
  DAC0/1 -> DAC Set/1(DAC0)
  DAC1/1 -> DAC Set/2(DAC1)
  DAC2/1 -> DAC Set/3(DAC2)
  DAC3/1 -> DAC Set/4(DAC3)
  DAC4/1 -> DAC Set/5(DAC4)
  DAC5/1 -> DAC Set/6(DAC5)
  DAC6/1 -> DAC Set/7(DAC6)
  DAC7/1 -> DAC Set/8(DAC7)
  RST/1 -> Byte Gen/4(In4), Byte Gen/6(In6), Byte Gen/8(In8), Byte Gen/10(In10), Byte Gen/12(In12), Byte Gen/14(In14), DAC Set/9(DAC_en), Byte Gen/16(In16), Byte Gen/2(In2)
  DAC Set/1(Out1) -> Packet Output1/4
  DAC Set/2(Out2) -> Packet Output1/5
  DAC Set/3(Out3) -> Packet Output1/6
  DAC Set/4(Out4) -> Packet Output1/7
  DAC Set/5(Out5) -> Packet Output1/8
  DAC Set/6(Out6) -> Packet Output1/9
  DAC Set/7(Out7) -> Packet Output1/10
  DAC Set/8(Out8) -> Packet Output1/11

== system Torque_Mode_OpenLoop/FUM SCARA/WRT_Target TSP MD Interface V2.0A/TEST RI ==
  DAC_in0 : Constant  Value=8
  DAC_in1 : Constant  Value=7
  DAC_in2 : Constant  Value=6
  DAC_in3 : Constant  Value=5
  DAC_in4 : Constant  Value=4
  DAC_in5 : Constant  Value=3
  DAC_in6 : Constant  Value=2
  DAC_in7 : Constant
  GPIO : Constant  Value=15  SampleTime=-1
  Rst : Constant  Value=0
  Out16 : Outport
  Out17 : Outport  Port=2
  Out18 : Outport  Port=3
  Out19 : Outport  Port=4
  Out20 : Outport  Port=5
  Out21 : Outport  Port=6
  Out22 : Outport  Port=7
  Out23 : Outport  Port=8
  Out24 : Outport  Port=9
  Out25 : Outport  Port=10
  wires:
  DAC_in4/1 -> Out21/1
  DAC_in6/1 -> Out23/1
  GPIO/1 -> Out25/1
  DAC_in1/1 -> Out18/1
  DAC_in3/1 -> Out20/1
  DAC_in2/1 -> Out19/1
  DAC_in0/1 -> Out17/1
  Rst/1 -> Out16/1
  DAC_in5/1 -> Out22/1
  DAC_in7/1 -> Out24/1

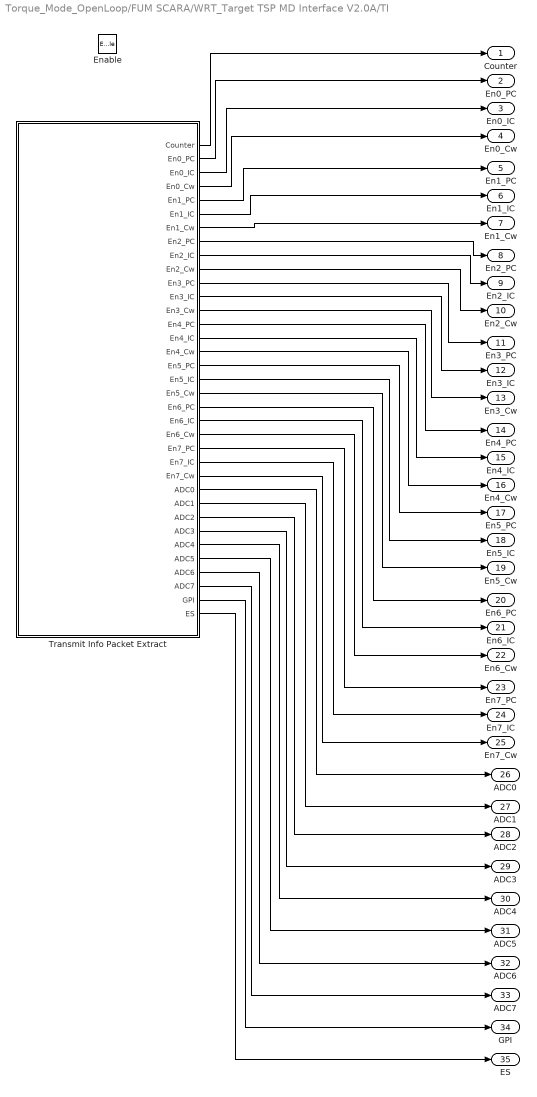
== system Torque_Mode_OpenLoop/FUM SCARA/WRT_Target TSP MD Interface V2.0A/TI ==
  Enable : EnablePort
  Transmit Info Packet Extract : Subsystem
  Counter : Outport
  En0_PC : Outport  Port=2
  En0_IC : Outport  Port=3
  En0_Cw : Outport  Port=4
  En1_PC : Outport  Port=5
  En1_IC : Outport  Port=6
  En1_Cw : Outport  Port=7
  En2_PC : Outport  Port=8
  En2_IC : Outport  Port=9
  En2_Cw : Outport  Port=10
  En3_PC : Outport  Port=11
  En3_IC : Outport  Port=12
  En3_Cw : Outport  Port=13
  En4_PC : Outport  Port=14
  En4_IC : Outport  Port=15
  En4_Cw : Outport  Port=16
  En5_PC : Outport  Port=17
  En5_IC : Outport  Port=18
  En5_Cw : Outport  Port=19
  En6_PC : Outport  Port=20
  En6_IC : Outport  Port=21
  En6_Cw : Outport  Port=22
  En7_PC : Outport  Port=23
  En7_IC : Outport  Port=24
  En7_Cw : Outport  Port=25
  ADC0 : Outport  Port=26
  ADC1 : Outport  Port=27
  ADC2 : Outport  Port=28
  ADC3 : Outport  Port=29
  ADC4 : Outport  Port=30
  ADC5 : Outport  Port=31
  ADC6 : Outport  Port=32
  ADC7 : Outport  Port=33
  GPI : Outport  Port=34
  ES : Outport  Port=35
  wires:
  Transmit Info Packet Extract/1(Counter) -> Counter/1
  Transmit Info Packet Extract/2(En0_PC) -> En0_PC/1
  Transmit Info Packet Extract/3(En0_IC) -> En0_IC/1
  Transmit Info Packet Extract/4(En0_Cw) -> En0_Cw/1
  Transmit Info Packet Extract/5(En1_PC) -> En1_PC/1
  Transmit Info Packet Extract/6(En1_IC) -> En1_IC/1
  Transmit Info Packet Extract/7(En1_Cw) -> En1_Cw/1
  Transmit Info Packet Extract/8(En2_PC) -> En2_PC/1
  Transmit Info Packet Extract/9(En2_IC) -> En2_IC/1
  Transmit Info Packet Extract/10(En2_Cw) -> En2_Cw/1
  Transmit Info Packet Extract/11(En3_PC) -> En3_PC/1
  Transmit Info Packet Extract/12(En3_IC) -> En3_IC/1
  Transmit Info Packet Extract/13(En3_Cw) -> En3_Cw/1
  Transmit Info Packet Extract/14(En4_PC) -> En4_PC/1
  Transmit Info Packet Extract/15(En4_IC) -> En4_IC/1
  Transmit Info Packet Extract/16(En4_Cw) -> En4_Cw/1
  Transmit Info Packet Extract/17(En5_PC) -> En5_PC/1
  Transmit Info Packet Extract/18(En5_IC) -> En5_IC/1
  Transmit Info Packet Extract/19(En5_Cw) -> En5_Cw/1
  Transmit Info Packet Extract/20(En6_PC) -> En6_PC/1
  Transmit Info Packet Extract/21(En6_IC) -> En6_IC/1
  Transmit Info Packet Extract/22(En6_Cw) -> En6_Cw/1
  Transmit Info Packet Extract/23(En7_PC) -> En7_PC/1
  Transmit Info Packet Extract/24(En7_IC) -> En7_IC/1
  Transmit Info Packet Extract/25(En7_Cw) -> En7_Cw/1
  Transmit Info Packet Extract/26(ADC0) -> ADC0/1
  Transmit Info Packet Extract/27(ADC1) -> ADC1/1
  Transmit Info Packet Extract/28(ADC2) -> ADC2/1
  Transmit Info Packet Extract/29(ADC3) -> ADC3/1
  Transmit Info Packet Extract/30(ADC4) -> ADC4/1
  Transmit Info Packet Extract/31(ADC5) -> ADC5/1
  Transmit Info Packet Extract/32(ADC6) -> ADC6/1
  Transmit Info Packet Extract/33(ADC7) -> ADC7/1
  Transmit Info Packet Extract/34(GPI) -> GPI/1
  Transmit Info Packet Extract/35(ES) -> ES/1

== system Torque_Mode_OpenLoop/FUM SCARA/WRT_Target TSP MD Interface V2.0A/TSP MDI Controller ==
  Constant1 : Constant  Value=MaxProcTime  SampleTime=-1
  Counter Limited : simulink/Sources/Counter Limited  uplimit=MaxProcTime  tsamp=SampleTime
  Data Type Conversion : DataTypeConversion
  TSP MDI Control State : Stateflow chart  TreatAsAtomicUnit=on
  StartStop En : Outport
  Rst Board : Outport  Port=2
  Process En : Outport  Port=3
  StopStart Setting : Outport  Port=4
  StateCounter : Outport  Port=5
  wires:
  Counter Limited/1 -> StateCounter/1, Data Type Conversion/1
  TSP MDI Control State/3(ProcessEn) -> Process En/1
  Constant1/1 -> TSP MDI Control State/2(MaxCounter)
  TSP MDI Control State/2(RstBoard) -> Rst Board/1
  TSP MDI Control State/1(StartStopEn) -> StartStop En/1
  TSP MDI Control State/4(StartStopSetting) -> StopStart Setting/1
  Data Type Conversion/1 -> TSP MDI Control State/1(CounterIn)

== system Torque_Mode_OpenLoop/FUM SCARA/WRT_Target TSP MD Interface V2.0A/MDI_Setting/Packet Gen ==
  Start/Stop : Inport
  Host Mac : Inport  Port=2
  Device Mac : Inport  Port=3
  Host Ip : Inport  Port=4
  Device Ip : Inport  Port=5
  Host Port : Inport  Port=6
  Device Port : Inport  Port=7
  Timer Interval : Inport  Port=8
  ADC Mode & Range : Inport  Port=9
  Constant1 : Constant
  Data Type Conversion{,1..10} (11 alike) : DataTypeConversion
  Packet Output : rtwinlib/Packet Output  SampleTime=SampleTime  MaxMissedTicks=1000  ShowMissedTicks=off  YieldWhenWaiting=on  DrvName=Standard_Devices/UDP_Protocol  DrvAddress=100  DrvOptions=[3232236031 101]  PacketSize=126  DataTypes={'126*uint8'}  ShowReady=off  ShowError=off  PacketID=1  ByteOrder=1  InitialValue=[]  FinalValue=[]
      settings: AttributesFormatString=Standard Devices\nUDP Protocol [64h]
  TimeGen : Subsystem
  Udp Setting : slrtlib/UDP/Pack   datatypes={'uint8','uint8','uint8','uint8','uint32','uint32','uint16','uint16','uint32','uint8','uint8'}  byteAlign=1
  Xml Header : Constant  Value=[60 63 120 109 108 32 118 101 114 115 105 111 110 61 34 49 46 48 34 63 62 60 116 115 112 105 115 104 114 111 62 60 116 121 112 101 62 77 68 73 95 115 101 116 116 105 110 103 60 47 116 121 112 101 62 60 115 105 122 101 62 51 48 60 47 115 105 122 101 62 60 118 97 108 117 101 62 ]  SampleTime=-1  LockScale=on
  Xml footer : Constant  Value=[60 47 118 97 108 117 101 62 60 47 116 115 112 105 115 104 114 111 62]  SampleTime=-1
  wires:
  Start/Stop/1 -> Data Type Conversion1/1
  Xml Header/1 -> Data Type Conversion/1
  Data Type Conversion/1 -> Udp Setting/1
  Host Mac/1 -> Data Type Conversion2/1
  Device Mac/1 -> Data Type Conversion3/1
  Host Ip/1 -> Data Type Conversion4/1
  Device Ip/1 -> Data Type Conversion5/1
  Host Port/1 -> Data Type Conversion6/1
  Device Port/1 -> Data Type Conversion7/1
  Timer Interval/1 -> TimeGen/1(value_time)
  ADC Mode & Range/1 -> Data Type Conversion8/1
  Data Type Conversion8/1 -> Udp Setting/10
  Xml footer/1 -> Data Type Conversion9/1
  Data Type Conversion9/1 -> Udp Setting/11
  Data Type Conversion2/1 -> Udp Setting/3
  Data Type Conversion3/1 -> Udp Setting/4
  Data Type Conversion4/1 -> Udp Setting/5
  Data Type Conversion5/1 -> Udp Setting/6
  Data Type Conversion6/1 -> Udp Setting/7
  Data Type Conversion7/1 -> Udp Setting/8
  Data Type Conversion10/1 -> Udp Setting/9
  Data Type Conversion1/1 -> Udp Setting/2
  TimeGen/1(Time_value) -> Data Type Conversion10/1
  Udp Setting/1 -> Packet Output/1

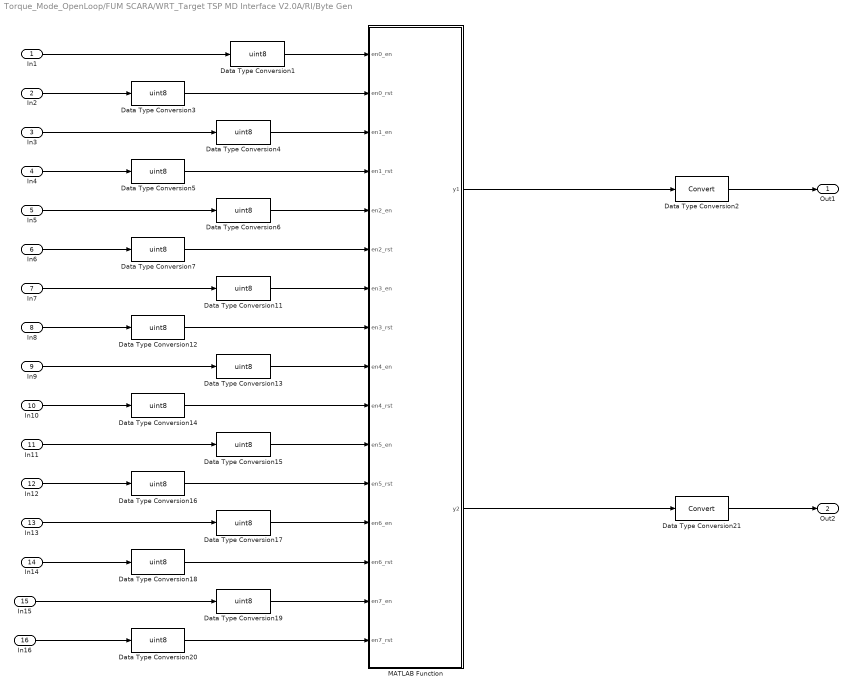
== system Torque_Mode_OpenLoop/FUM SCARA/WRT_Target TSP MD Interface V2.0A/RI/Byte Gen ==
  In1 : Inport
  In2 : Inport  Port=2
  In3 : Inport  Port=3
  In4 : Inport  Port=4
  In5 : Inport  Port=5
  In6 : Inport  Port=6
  In7 : Inport  Port=7
  In8 : Inport  Port=8
  In9 : Inport  Port=9
  In10 : Inport  Port=10
  In11 : Inport  Port=11
  In12 : Inport  Port=12
  In13 : Inport  Port=13
  In14 : Inport  Port=14
  In15 : Inport  Port=15
  In16 : Inport  Port=16
  Data Type Conversion{1,3..7,11..20} (16 alike) : DataTypeConversion  OutDataTypeStr=uint8
  Data Type Conversion2 : DataTypeConversion
  Data Type Conversion21 : DataTypeConversion
  MATLAB Function : MATLAB Function  TreatAsAtomicUnit=on
  Out1 : Outport
  Out2 : Outport  Port=2
  wires:
  In2/1 -> Data Type Conversion3/1
  Data Type Conversion21/1 -> Out2/1
  Data Type Conversion20/1 -> MATLAB Function/16(en7_rst)
  MATLAB Function/1(y1) -> Data Type Conversion2/1
  In11/1 -> Data Type Conversion15/1
  Data Type Conversion15/1 -> MATLAB Function/11(en5_en)
  In14/1 -> Data Type Conversion18/1
  In5/1 -> Data Type Conversion6/1
  Data Type Conversion17/1 -> MATLAB Function/13(en6_en)
  MATLAB Function/2(y2) -> Data Type Conversion21/1
  Data Type Conversion16/1 -> MATLAB Function/12(en5_rst)
  Data Type Conversion18/1 -> MATLAB Function/14(en6_rst)
  Data Type Conversion19/1 -> MATLAB Function/15(en7_en)
  Data Type Conversion1/1 -> MATLAB Function/1(en0_en)
  In10/1 -> Data Type Conversion14/1
  Data Type Conversion11/1 -> MATLAB Function/7(en3_en)
  Data Type Conversion5/1 -> MATLAB Function/4(en1_rst)
  In6/1 -> Data Type Conversion7/1
  Data Type Conversion6/1 -> MATLAB Function/5(en2_en)
  In15/1 -> Data Type Conversion19/1
  In16/1 -> Data Type Conversion20/1
  Data Type Conversion12/1 -> MATLAB Function/8(en3_rst)
  Data Type Conversion4/1 -> MATLAB Function/3(en1_en)
  In9/1 -> Data Type Conversion13/1
  Data Type Conversion7/1 -> MATLAB Function/6(en2_rst)
  Data Type Conversion3/1 -> MATLAB Function/2(en0_rst)
  In4/1 -> Data Type Conversion5/1
  In13/1 -> Data Type Conversion17/1
  In7/1 -> Data Type Conversion11/1
  In8/1 -> Data Type Conversion12/1
  In12/1 -> Data Type Conversion16/1
  In3/1 -> Data Type Conversion4/1
  Data Type Conversion14/1 -> MATLAB Function/10(en4_rst)
  Data Type Conversion13/1 -> MATLAB Function/9(en4_en)
  In1/1 -> Data Type Conversion1/1
  Data Type Conversion2/1 -> Out1/1

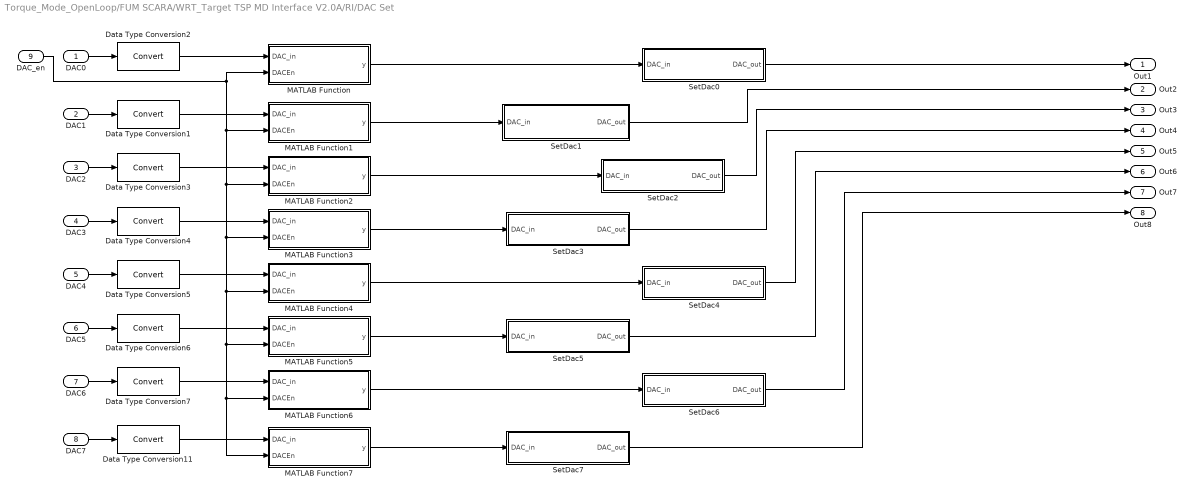
== system Torque_Mode_OpenLoop/FUM SCARA/WRT_Target TSP MD Interface V2.0A/RI/DAC Set ==
  DAC0 : Inport
  DAC1 : Inport  Port=2
  DAC2 : Inport  Port=3
  DAC3 : Inport  Port=4
  DAC4 : Inport  Port=5
  DAC5 : Inport  Port=6
  DAC6 : Inport  Port=7
  DAC7 : Inport  Port=8
  DAC_en : Inport  Port=9
  Data Type Conversion{1..7,11} (8 alike) : DataTypeConversion
  MATLAB Function : MATLAB Function  TreatAsAtomicUnit=on
  MATLAB Function1 : MATLAB Function  TreatAsAtomicUnit=on
  MATLAB Function2 : MATLAB Function  TreatAsAtomicUnit=on
  MATLAB Function3 : MATLAB Function  TreatAsAtomicUnit=on
  MATLAB Function4 : MATLAB Function  TreatAsAtomicUnit=on
  MATLAB Function5 : MATLAB Function  TreatAsAtomicUnit=on
  MATLAB Function6 : MATLAB Function  TreatAsAtomicUnit=on
  MATLAB Function7 : MATLAB Function  TreatAsAtomicUnit=on
  SetDac0 : Subsystem
  SetDac1 : Subsystem
  SetDac2 : Subsystem
  SetDac3 : Subsystem
  SetDac4 : Subsystem
  SetDac5 : Subsystem
  SetDac6 : Subsystem
  SetDac7 : Subsystem
  Out1 : Outport
  Out2 : Outport  Port=2
  Out3 : Outport  Port=3
  Out4 : Outport  Port=4
  Out5 : Outport  Port=5
  Out6 : Outport  Port=6
  Out7 : Outport  Port=7
  Out8 : Outport  Port=8
  wires:
  Data Type Conversion4/1 -> MATLAB Function3/1(DAC_in)
  SetDac0/1(DAC_out) -> Out1/1
  SetDac1/1(DAC_out) -> Out2/1
  SetDac2/1(DAC_out) -> Out3/1
  SetDac3/1(DAC_out) -> Out4/1
  SetDac4/1(DAC_out) -> Out5/1
  SetDac5/1(DAC_out) -> Out6/1
  SetDac6/1(DAC_out) -> Out7/1
  SetDac7/1(DAC_out) -> Out8/1
  MATLAB Function6/1(y) -> SetDac6/1(DAC_in)
  DAC4/1 -> Data Type Conversion5/1
  DAC3/1 -> Data Type Conversion4/1
  DAC7/1 -> Data Type Conversion11/1
  MATLAB Function1/1(y) -> SetDac1/1(DAC_in)
  MATLAB Function4/1(y) -> SetDac4/1(DAC_in)
  DAC6/1 -> Data Type Conversion7/1
  DAC1/1 -> Data Type Conversion1/1
  MATLAB Function7/1(y) -> SetDac7/1(DAC_in)
  DAC_en/1 -> MATLAB Function/2(DACEn), MATLAB Function1/2(DACEn), MATLAB Function2/2(DACEn), MATLAB Function3/2(DACEn), MATLAB Function4/2(DACEn), MATLAB Function5/2(DACEn), MATLAB Function6/2(DACEn), MATLAB Function7/2(DACEn)
  DAC2/1 -> Data Type Conversion3/1
  MATLAB Function5/1(y) -> SetDac5/1(DAC_in)
  MATLAB Function3/1(y) -> SetDac3/1(DAC_in)
  DAC5/1 -> Data Type Conversion6/1
  Data Type Conversion1/1 -> MATLAB Function1/1(DAC_in)
  Data Type Conversion6/1 -> MATLAB Function5/1(DAC_in)
  MATLAB Function/1(y) -> SetDac0/1(DAC_in)
  MATLAB Function2/1(y) -> SetDac2/1(DAC_in)
  Data Type Conversion11/1 -> MATLAB Function7/1(DAC_in)
  Data Type Conversion2/1 -> MATLAB Function/1(DAC_in)
  Data Type Conversion5/1 -> MATLAB Function4/1(DAC_in)
  Data Type Conversion7/1 -> MATLAB Function6/1(DAC_in)
  Data Type Conversion3/1 -> MATLAB Function2/1(DAC_in)
  DAC0/1 -> Data Type Conversion2/1

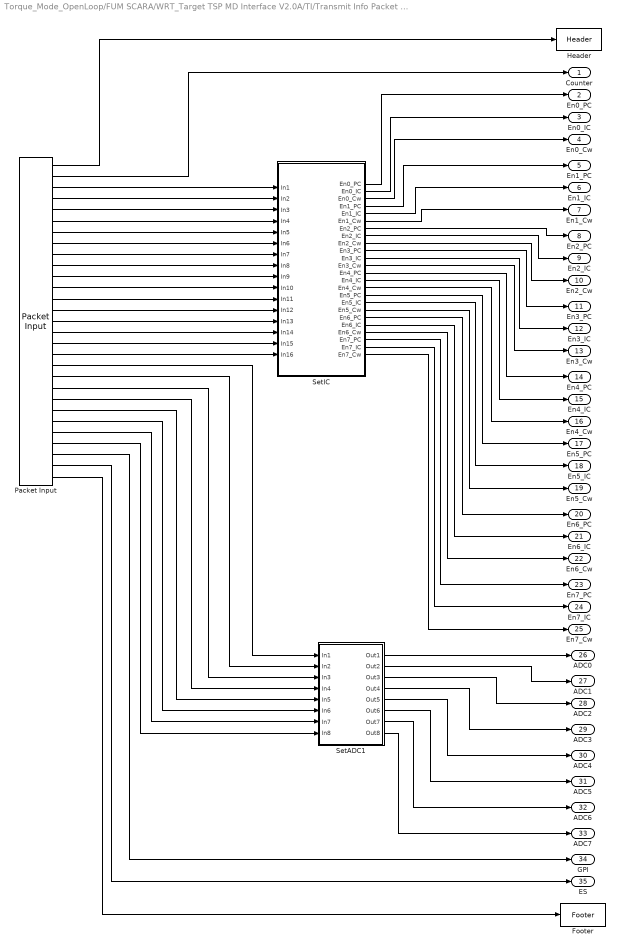
== system Torque_Mode_OpenLoop/FUM SCARA/WRT_Target TSP MD Interface V2.0A/TI/Transmit Info Packet Extract ==
  Footer : ToWorkspace  VariableName=Footer  SaveFormat=Timeseries  SampleTime=-1
  Header : ToWorkspace  VariableName=Header  SaveFormat=Timeseries  SampleTime=-1
  Packet Input : rtwinlib/Packet Input  SampleTime=SampleTime  MaxMissedTicks=1000  ShowMissedTicks=off  YieldWhenWaiting=on  DrvName=Standard_Devices/UDP_Protocol  DrvAddress=23000  DrvOptions=[3232235798 23001]  PacketSize=186  DataTypes="{'81*uint8' 'uint8' 'int32' 'uint32' 'int32' 'uint32' 'int32' 'uint32' 'int32' 'uint32' 'int32' 'uint32' 'int32' 'uint32' 'int32' 'uint32' 'int32' 'uint32' 'int16' 'int16' 'int16' 'int16' 'int16' 'int16' 'int16' 'int16' 'uint32'  'uint8' '19*uint8'}"  ShowReady=off  ShowError=off  PacketID=1  ByteOrder=1  ShowTimestamp=off
      settings: AttributesFormatString=Standard Devices\nUDP Protocol [59D8h]
  SetADC1 : Subsystem
  SetIC : Subsystem
  Counter : Outport
  En0_PC : Outport  Port=2
  En0_IC : Outport  Port=3
  En0_Cw : Outport  Port=4
  En1_PC : Outport  Port=5
  En1_IC : Outport  Port=6
  En1_Cw : Outport  Port=7
  En2_PC : Outport  Port=8
  En2_IC : Outport  Port=9
  En2_Cw : Outport  Port=10
  En3_PC : Outport  Port=11
  En3_IC : Outport  Port=12
  En3_Cw : Outport  Port=13
  En4_PC : Outport  Port=14
  En4_IC : Outport  Port=15
  En4_Cw : Outport  Port=16
  En5_PC : Outport  Port=17
  En5_IC : Outport  Port=18
  En5_Cw : Outport  Port=19
  En6_PC : Outport  Port=20
  En6_IC : Outport  Port=21
  En6_Cw : Outport  Port=22
  En7_PC : Outport  Port=23
  En7_IC : Outport  Port=24
  En7_Cw : Outport  Port=25
  ADC0 : Outport  Port=26
  ADC1 : Outport  Port=27
  ADC2 : Outport  Port=28
  ADC3 : Outport  Port=29
  ADC4 : Outport  Port=30
  ADC5 : Outport  Port=31
  ADC6 : Outport  Port=32
  ADC7 : Outport  Port=33
  GPI : Outport  Port=34
  ES : Outport  Port=35
  wires:
  Packet Input/1 -> Header/1
  Packet Input/26 -> SetADC1/8(In8)
  Packet Input/25 -> SetADC1/7(In7)
  Packet Input/24 -> SetADC1/6(In6)
  Packet Input/23 -> SetADC1/5(In5)
  Packet Input/22 -> SetADC1/4(In4)
  Packet Input/21 -> SetADC1/3(In3)
  Packet Input/20 -> SetADC1/2(In2)
  Packet Input/19 -> SetADC1/1(In1)
  Packet Input/2 -> Counter/1
  SetADC1/8(Out8) -> ADC7/1
  SetADC1/7(Out7) -> ADC6/1
  SetADC1/6(Out6) -> ADC5/1
  SetADC1/5(Out5) -> ADC4/1
  SetADC1/4(Out4) -> ADC3/1
  SetADC1/3(Out3) -> ADC2/1
  SetADC1/2(Out2) -> ADC1/1
  SetADC1/1(Out1) -> ADC0/1
  Packet Input/27 -> GPI/1
  Packet Input/3 -> SetIC/1(In1)
  Packet Input/4 -> SetIC/2(In2)
  Packet Input/5 -> SetIC/3(In3)
  Packet Input/6 -> SetIC/4(In4)
  Packet Input/7 -> SetIC/5(In5)
  Packet Input/8 -> SetIC/6(In6)
  Packet Input/9 -> SetIC/7(In7)
  Packet Input/10 -> SetIC/8(In8)
  Packet Input/11 -> SetIC/9(In9)
  Packet Input/12 -> SetIC/10(In10)
  Packet Input/13 -> SetIC/11(In11)
  Packet Input/14 -> SetIC/12(In12)
  Packet Input/15 -> SetIC/13(In13)
  Packet Input/16 -> SetIC/14(In14)
  Packet Input/17 -> SetIC/15(In15)
  Packet Input/18 -> SetIC/16(In16)
  SetIC/1(En0_PC) -> En0_PC/1
  SetIC/2(En0_IC) -> En0_IC/1
  SetIC/3(En0_Cw) -> En0_Cw/1
  SetIC/4(En1_PC) -> En1_PC/1
  SetIC/5(En1_IC) -> En1_IC/1
  SetIC/6(En1_Cw) -> En1_Cw/1
  SetIC/7(En2_PC) -> En2_PC/1
  SetIC/8(En2_IC) -> En2_IC/1
  SetIC/9(En2_Cw) -> En2_Cw/1
  SetIC/10(En3_PC) -> En3_PC/1
  SetIC/11(En3_IC) -> En3_IC/1
  SetIC/12(En3_Cw) -> En3_Cw/1
  SetIC/13(En4_PC) -> En4_PC/1
  SetIC/14(En4_IC) -> En4_IC/1
  SetIC/15(En4_Cw) -> En4_Cw/1
  SetIC/16(En5_PC) -> En5_PC/1
  SetIC/17(En5_IC) -> En5_IC/1
  SetIC/18(En5_Cw) -> En5_Cw/1
  SetIC/19(En6_PC) -> En6_PC/1
  SetIC/20(En6_IC) -> En6_IC/1
  SetIC/21(En6_Cw) -> En6_Cw/1
  SetIC/22(En7_PC) -> En7_PC/1
  SetIC/23(En7_IC) -> En7_IC/1
  SetIC/24(En7_Cw) -> En7_Cw/1
  Packet Input/29 -> Footer/1
  Packet Input/28 -> ES/1

== system Torque_Mode_OpenLoop/FUM SCARA/WRT_Target TSP MD Interface V2.0A/MDI_Setting/Packet Gen/TimeGen ==
  value_time : Inport
  Constant : Constant  Value=100  SampleTime=-1
  Product : Product
  Time_value : Outport
  wires:
  value_time/1 -> Product/1
  Product/1 -> Time_value/1
  Constant/1 -> Product/2

== system Torque_Mode_OpenLoop/FUM SCARA/WRT_Target TSP MD Interface V2.0A/RI/DAC Set/SetDac0 ==
  DAC_in : Inport
  Add : Sum
  Data Type Conversion0 : DataTypeConversion
  Divide : Product  Inputs=*/
  Divide_numb : Constant  Value=20
  FFFF_numb : Constant  Value=65535
  Product : Product
  Product_numb : Constant  Value=10
  DAC_out : Outport
  wires:
  Divide_numb/1 -> Divide/2
  Product/1 -> Divide/1
  Divide/1 -> Data Type Conversion0/1
  Product_numb/1 -> Add/2
  FFFF_numb/1 -> Product/2
  Add/1 -> Product/1
  DAC_in/1 -> Add/1
  Data Type Conversion0/1 -> DAC_out/1

== system Torque_Mode_OpenLoop/FUM SCARA/WRT_Target TSP MD Interface V2.0A/RI/DAC Set/SetDac1 ==
  DAC_in : Inport
  Add : Sum
  Data Type Conversion0 : DataTypeConversion
  Divide : Product  Inputs=*/
  Divide_numb : Constant  Value=20
  FFFF_numb : Constant  Value=65535
  Product : Product
  Product_numb : Constant  Value=10
  DAC_out : Outport
  wires:
  Divide_numb/1 -> Divide/2
  Product/1 -> Divide/1
  Divide/1 -> Data Type Conversion0/1
  Product_numb/1 -> Add/2
  FFFF_numb/1 -> Product/2
  Add/1 -> Product/1
  DAC_in/1 -> Add/1
  Data Type Conversion0/1 -> DAC_out/1

== system Torque_Mode_OpenLoop/FUM SCARA/WRT_Target TSP MD Interface V2.0A/RI/DAC Set/SetDac2 ==
  DAC_in : Inport
  Add : Sum
  Data Type Conversion0 : DataTypeConversion
  Divide : Product  Inputs=*/
  Divide_numb : Constant  Value=20
  FFFF_numb : Constant  Value=65535
  Product : Product
  Product_numb : Constant  Value=10
  DAC_out : Outport
  wires:
  Divide_numb/1 -> Divide/2
  Product/1 -> Divide/1
  Divide/1 -> Data Type Conversion0/1
  Product_numb/1 -> Add/2
  FFFF_numb/1 -> Product/2
  Add/1 -> Product/1
  DAC_in/1 -> Add/1
  Data Type Conversion0/1 -> DAC_out/1

== system Torque_Mode_OpenLoop/FUM SCARA/WRT_Target TSP MD Interface V2.0A/RI/DAC Set/SetDac3 ==
  DAC_in : Inport
  Add : Sum
  Data Type Conversion0 : DataTypeConversion
  Divide : Product  Inputs=*/
  Divide_numb : Constant  Value=20
  FFFF_numb : Constant  Value=65535
  Product : Product
  Product_numb : Constant  Value=10
  DAC_out : Outport
  wires:
  Divide_numb/1 -> Divide/2
  Product/1 -> Divide/1
  Divide/1 -> Data Type Conversion0/1
  Product_numb/1 -> Add/2
  FFFF_numb/1 -> Product/2
  Add/1 -> Product/1
  DAC_in/1 -> Add/1
  Data Type Conversion0/1 -> DAC_out/1

== system Torque_Mode_OpenLoop/FUM SCARA/WRT_Target TSP MD Interface V2.0A/RI/DAC Set/SetDac4 ==
  DAC_in : Inport
  Add : Sum
  Data Type Conversion0 : DataTypeConversion
  Divide : Product  Inputs=*/
  Divide_numb : Constant  Value=20
  FFFF_numb : Constant  Value=65535
  Product : Product
  Product_numb : Constant  Value=10
  DAC_out : Outport
  wires:
  Divide_numb/1 -> Divide/2
  Product/1 -> Divide/1
  Divide/1 -> Data Type Conversion0/1
  Product_numb/1 -> Add/2
  FFFF_numb/1 -> Product/2
  Add/1 -> Product/1
  DAC_in/1 -> Add/1
  Data Type Conversion0/1 -> DAC_out/1

== system Torque_Mode_OpenLoop/FUM SCARA/WRT_Target TSP MD Interface V2.0A/RI/DAC Set/SetDac5 ==
  DAC_in : Inport
  Add : Sum
  Data Type Conversion0 : DataTypeConversion
  Divide : Product  Inputs=*/
  Divide_numb : Constant  Value=20
  FFFF_numb : Constant  Value=65535
  Product : Product
  Product_numb : Constant  Value=10
  DAC_out : Outport
  wires:
  Divide_numb/1 -> Divide/2
  Product/1 -> Divide/1
  Divide/1 -> Data Type Conversion0/1
  Product_numb/1 -> Add/2
  FFFF_numb/1 -> Product/2
  Add/1 -> Product/1
  DAC_in/1 -> Add/1
  Data Type Conversion0/1 -> DAC_out/1

== system Torque_Mode_OpenLoop/FUM SCARA/WRT_Target TSP MD Interface V2.0A/RI/DAC Set/SetDac6 ==
  DAC_in : Inport
  Add : Sum
  Data Type Conversion0 : DataTypeConversion
  Divide : Product  Inputs=*/
  Divide_numb : Constant  Value=20
  FFFF_numb : Constant  Value=65535
  Product : Product
  Product_numb : Constant  Value=10
  DAC_out : Outport
  wires:
  Divide_numb/1 -> Divide/2
  Product/1 -> Divide/1
  Divide/1 -> Data Type Conversion0/1
  Product_numb/1 -> Add/2
  FFFF_numb/1 -> Product/2
  Add/1 -> Product/1
  DAC_in/1 -> Add/1
  Data Type Conversion0/1 -> DAC_out/1

== system Torque_Mode_OpenLoop/FUM SCARA/WRT_Target TSP MD Interface V2.0A/RI/DAC Set/SetDac7 ==
  DAC_in : Inport
  Add : Sum
  Data Type Conversion0 : DataTypeConversion
  Divide : Product  Inputs=*/
  Divide_numb : Constant  Value=20
  FFFF_numb : Constant  Value=65535
  Product : Product
  Product_numb : Constant  Value=10
  DAC_out : Outport
  wires:
  Divide_numb/1 -> Divide/2
  Product/1 -> Divide/1
  Divide/1 -> Data Type Conversion0/1
  Product_numb/1 -> Add/2
  FFFF_numb/1 -> Product/2
  Add/1 -> Product/1
  DAC_in/1 -> Add/1
  Data Type Conversion0/1 -> DAC_out/1

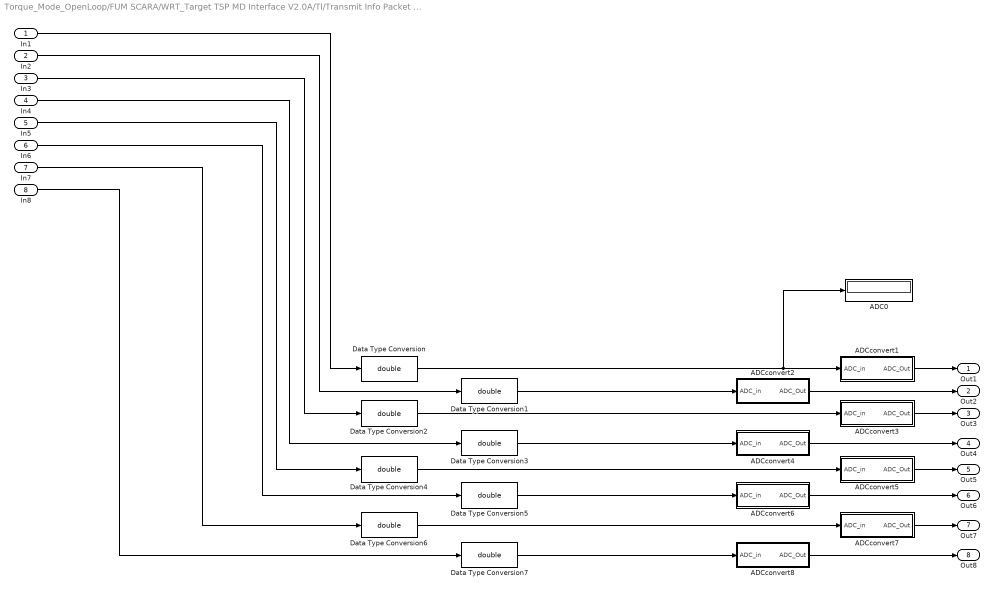
== system Torque_Mode_OpenLoop/FUM SCARA/WRT_Target TSP MD Interface V2.0A/TI/Transmit Info Packet Extract/SetADC1 ==
  In1 : Inport
  In2 : Inport  Port=2
  In3 : Inport  Port=3
  In4 : Inport  Port=4
  In5 : Inport  Port=5
  In6 : Inport  Port=6
  In7 : Inport  Port=7
  In8 : Inport  Port=8
  ADC0 : Display
  ADCconvert1 : Subsystem
  ADCconvert2 : Subsystem
  ADCconvert3 : Subsystem
  ADCconvert4 : Subsystem
  ADCconvert5 : Subsystem
  ADCconvert6 : Subsystem
  ADCconvert7 : Subsystem
  ADCconvert8 : Subsystem
  Data Type Conversion{,1..7} (8 alike) : DataTypeConversion  OutDataTypeStr=double
  Out1 : Outport
  Out2 : Outport  Port=2
  Out3 : Outport  Port=3
  Out4 : Outport  Port=4
  Out5 : Outport  Port=5
  Out6 : Outport  Port=6
  Out7 : Outport  Port=7
  Out8 : Outport  Port=8
  wires:
  In1/1 -> Data Type Conversion/1
  ADCconvert2/1(ADC_Out) -> Out2/1
  ADCconvert1/1(ADC_Out) -> Out1/1
  In2/1 -> Data Type Conversion1/1
  In3/1 -> Data Type Conversion2/1
  In4/1 -> Data Type Conversion3/1
  In5/1 -> Data Type Conversion4/1
  In6/1 -> Data Type Conversion5/1
  In7/1 -> Data Type Conversion6/1
  In8/1 -> Data Type Conversion7/1
  ADCconvert3/1(ADC_Out) -> Out3/1
  ADCconvert4/1(ADC_Out) -> Out4/1
  ADCconvert5/1(ADC_Out) -> Out5/1
  ADCconvert6/1(ADC_Out) -> Out6/1
  ADCconvert7/1(ADC_Out) -> Out7/1
  ADCconvert8/1(ADC_Out) -> Out8/1
  Data Type Conversion/1 -> ADCconvert1/1(ADC_in), ADC0/1
  Data Type Conversion2/1 -> ADCconvert3/1(ADC_in)
  Data Type Conversion1/1 -> ADCconvert2/1(ADC_in)
  Data Type Conversion3/1 -> ADCconvert4/1(ADC_in)
  Data Type Conversion4/1 -> ADCconvert5/1(ADC_in)
  Data Type Conversion5/1 -> ADCconvert6/1(ADC_in)
  Data Type Conversion6/1 -> ADCconvert7/1(ADC_in)
  Data Type Conversion7/1 -> ADCconvert8/1(ADC_in)
